simulink model "SMO_conventional"  (R2019b)
settings: Solver=VariableStepAuto  StartTime=0.0  StopTime=1  RelTol=1e-3
InitFcn:
  | run('MotorParamInit_1_5PMSM.m');
StopFcn:
  | %run('Calc_We_ThetaErr_Estimate_Harmonics.m');
values from neighbouring files (symbols this model uses):
  Ibase = 2*Pbase/Vbase/3    [MotorParamInit_1_5PMSM.m]
  J = 0.01    [MotorParamInit_1_5PMSM.m]
  KiPLL = 2*pi*fPIPLL*KpPLL    (= 209.439510239)    [MotorParamInit_1_5PMSM.m]
  KpCRd = 1.04    [MotorParamInit_1_5PMSM.m]
  KpCRq = 1.04    [MotorParamInit_1_5PMSM.m]
  KpPLL = 2*pi*fcutPLL/Webase    (= 1.66666666667)    [MotorParamInit_1_5PMSM.m]
  KpSR = 5.51    [MotorParamInit_1_5PMSM.m]
  Ld = 65.13e-3    (= 0.06513)    [MotorParamInit_1_5PMSM.m]
  LdPU = Ld/Lbase    [MotorParamInit_1_5PMSM.m]
  Lq = 120e-3    (= 0.12)    [MotorParamInit_1_5PMSM.m]
  LqPU = Lq/Lbase    [MotorParamInit_1_5PMSM.m]
  Np = 2    [MotorParamInit_1_5PMSM.m]
  PhifPU = Phif/Phibase    [MotorParamInit_1_5PMSM.m]
  Rs = 6.569    [MotorParamInit_1_5PMSM.m]
  RsPU = Rs/Zbase    [MotorParamInit_1_5PMSM.m]
  TaoiCRd = 4e-3    (= 0.004)    [MotorParamInit_1_5PMSM.m]
  TaoiCRq = 4e-3    (= 0.004)    [MotorParamInit_1_5PMSM.m]
  TaoiSR = 80e-3    (= 0.08)    [MotorParamInit_1_5PMSM.m]
  TaoLPF = 1/fLPF/2/pi    (= 0.00159154943092)    [MotorParamInit_1_5PMSM.m]
  Tctrl = 1/fctrl    (= 0.0001)    [MotorParamInit_1_5PMSM.m]
  TctrlPU = Tctrl/Tbase    (= 0.0376991118431)    [MotorParamInit_1_5PMSM.m]
  Tembase = Pbase/Wmbase    (= 7.95774715459)    [MotorParamInit_1_5PMSM.m]
  Ts = 1e-6    (= 1e-06)    [MotorParamInit_1_5PMSM.m]
  Vbase = VN*sqrt(2)/sqrt(3)    [MotorParamInit_1_5PMSM.m]
  Webase = 2*pi*fN    (= 376.991118431)    [MotorParamInit_1_5PMSM.m]
  Wmbase = Webase/Np    (= 188.495559215)    [MotorParamInit_1_5PMSM.m]
undefined symbols (not defined in the file or in its folder): DiscIntNeverNeededParam
libraries: simulink x6, powerlib x5, powerlib_extras x1
settings Model: Creator=W002220B  LastModifiedBy=W002220B

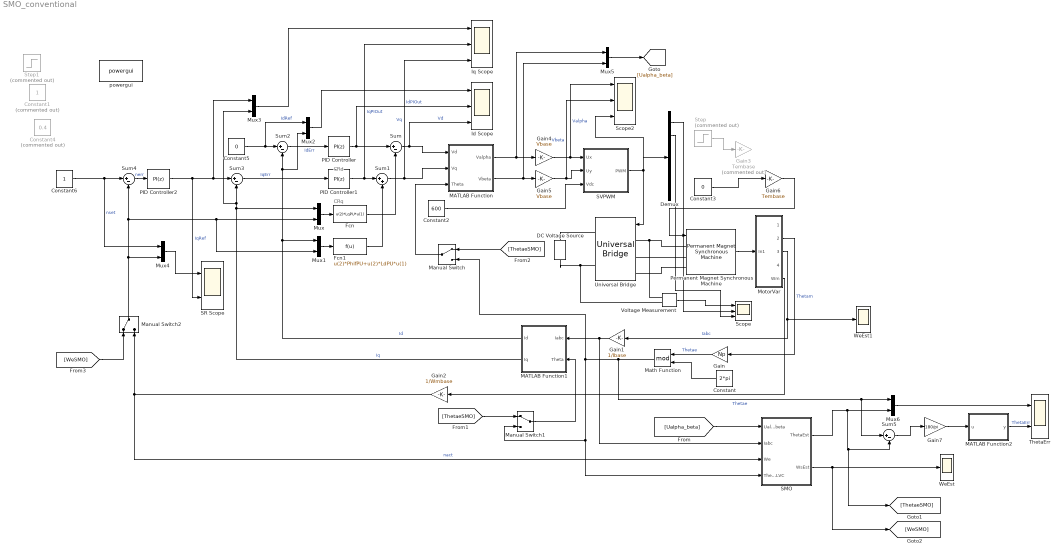
== system SMO_conventional ==
  note: CRd
  note: CRq
  Constant : Constant  Value=2*pi
  Constant1 : Constant  Commented=on
  Constant2 : Constant  Value=600
  Constant3 : Constant  Value=0
  Constant4 : Constant  Commented=on  Value=0.4
  Constant5 : Constant  Value=0
  Constant6 : Constant
  DC Voltage Source : powerlib/Electrical Sources/DC Voltage Source  Amplitude=600  Measurements=None
      settings: SourceProductName=Simscape Electrical
  Demux : Demux  Outputs=6
  Fcn : Fcn  Expr=u(2)*LqPU*u(1)
  Fcn1 : Fcn  Expr=u(2)*PhifPU+u(2)*LdPU*u(1)
  Gain : Gain  Gain=Np
  Gain1 : Gain  Gain=1/Ibase
  Gain2 : Gain  Gain=1/Wmbase
  Gain3 : Gain  Commented=on  Gain=Tembase
  Gain4 : Gain  Gain=Vbase
  Gain5 : Gain  Gain=Vbase
  Gain6 : Gain  Gain=Tembase
  Gain7 : Gain  Gain=180/pi
  Id Scope : Scope  NumInputPorts=3
  Iq Scope : Scope  NumInputPorts=3
  MATLAB Function : MATLAB Function  TreatAsAtomicUnit=on
  MATLAB Function1 : MATLAB Function  TreatAsAtomicUnit=on
  MATLAB Function2 : MATLAB Function  TreatAsAtomicUnit=on
  Manual Switch : ManualSwitch
  Manual Switch1 : ManualSwitch
  Manual Switch2 : ManualSwitch
  Math Function : Math  Operator=mod  SignedPower=off  SaturateOnIntegerOverflow=on
  MotorVar : Subsystem
  Mux{,1..6} (7 alike) : Mux  Inputs=2
  PID Controller : simulink/Continuous/PID Controller  Controller=PI  Form=Parallel  TimeDomain=Discrete-time  SampleTime=Tctrl  IntegratorMethod=Forward Euler  FilterMethod=Forward Euler  ControllerParametersSource=internal  P=KpCRd  I=KpCRd/TaoiCRd  D=0  UseFilter=on  N=100  TunerSelectOption=Transfer Function Based (PID Tuner App)  InitialConditionSource=internal  InitialConditionForIntegrator=0  InitialConditionForFilter=0  DifferentiatorICPrevScaledInput=0  ExternalReset=none  TrackingMode=off  Kt=1  LimitOutput=on  UpperSaturationLimit=0.5  LowerSaturationLimit=-0.5  LinearizeAsGain=on  AntiWindupMode=clamping  Kb=1  POutMin=[]  POutMax=[]  IOutMin=[]  IOutMax=[]  DOutMin=[]  DOutMax=[]  NOutMin=[]  NOutMax=[]  SumOutMin=[]  SumOutMax=[]  SaturationOutMin=[]  SaturationOutMax=[]  PParamMin=[]  PParamMax=[]  IParamMin=[]  IParamMax=[]  DParamMin=[]  DParamMax=[]  NParamMin=[]  NParamMax=[]  KbParamMin=[]  KbParamMax=[]  KtParamMin=[]  KtParamMax=[]  KbOutMin=[]  KbOutMax=[]  KtOutMin=[]  KtOutMax=[]  IntegratorOutMin=[]  IntegratorOutMax=[]  FilterOutMin=[]  FilterOutMax=[]  SumI1OutMin=[]  SumI1OutMax=[]  SumI2OutMin=[]  SumI2OutMax=[]  SumI3OutMin=[]  SumI3OutMax=[]  SumI4OutMin=[]  SumI4OutMax=[]  SumDOutMin=[]  SumDOutMax=[]  DifferentiatorOutMin=[]  DifferentiatorOutMax=[]  FilterDiffOutCoefMin=[]  FilterDiffOutCoefMax=[]  ReciprocalOutMin=[]  ReciprocalOutMax=[]  SumDenOutMin=[]  SumDenOutMax=[]  SumNumOutMin=[]  SumNumOutMax=[]  DivideOutMin=[]  DivideOutMax=[]  IntegratorContinuousStateAttributes=''  IntegratorStateMustResolveToSignalObject=off  IntegratorRTWStateStorageClass=Auto  FilterContinuousStateAttributes=''  FilterStateMustResolveToSignalObject=off  FilterRTWStateStorageClass=Auto  ParallelPVariant=InternalParameters  IdealPVariant=Disabled  IVariant=InternalParameters  DVariant=Disabled  IntegratorVariant=Discrete  SatVariant=Enabled  AWVariant=DiscClampingParallel  PCopyVariant=Disabled  TRVariant=Disabled  FdbkBlocksVariant=Forward  IdealPFdbkVariant=Disabled  SatFdbkVariant=Disabled  DerivativeFilterVariant=Disabled  NVariant=Disabled  NCopyVariant=Disabled_SignalSpec  FilterICVariant=Disabled  IntegratorICVariant=InternalICs  ExternalResetVariant=Disabled  TRSumVariant=Passthrough  SumFdbkVariant=Disabled  SumVariant=Sum_PI
  PID Controller1 : simulink/Continuous/PID Controller  Controller=PI  Form=Parallel  TimeDomain=Discrete-time  SampleTime=Tctrl  IntegratorMethod=Forward Euler  FilterMethod=Forward Euler  ControllerParametersSource=internal  P=KpCRq  I=KpCRq/TaoiCRq  D=0  UseFilter=on  N=100  TunerSelectOption=Transfer Function Based (PID Tuner App)  InitialConditionSource=internal  InitialConditionForIntegrator=0  InitialConditionForFilter=0  DifferentiatorICPrevScaledInput=0  ExternalReset=none  TrackingMode=off  Kt=1  LimitOutput=on  UpperSaturationLimit=0.5  LowerSaturationLimit=-0.5  LinearizeAsGain=on  AntiWindupMode=clamping  Kb=1  POutMin=[]  POutMax=[]  IOutMin=[]  IOutMax=[]  DOutMin=[]  DOutMax=[]  NOutMin=[]  NOutMax=[]  SumOutMin=[]  SumOutMax=[]  SaturationOutMin=[]  SaturationOutMax=[]  PParamMin=[]  PParamMax=[]  IParamMin=[]  IParamMax=[]  DParamMin=[]  DParamMax=[]  NParamMin=[]  NParamMax=[]  KbParamMin=[]  KbParamMax=[]  KtParamMin=[]  KtParamMax=[]  KbOutMin=[]  KbOutMax=[]  KtOutMin=[]  KtOutMax=[]  IntegratorOutMin=[]  IntegratorOutMax=[]  FilterOutMin=[]  FilterOutMax=[]  SumI1OutMin=[]  SumI1OutMax=[]  SumI2OutMin=[]  SumI2OutMax=[]  SumI3OutMin=[]  SumI3OutMax=[]  SumI4OutMin=[]  SumI4OutMax=[]  SumDOutMin=[]  SumDOutMax=[]  DifferentiatorOutMin=[]  DifferentiatorOutMax=[]  FilterDiffOutCoefMin=[]  FilterDiffOutCoefMax=[]  ReciprocalOutMin=[]  ReciprocalOutMax=[]  SumDenOutMin=[]  SumDenOutMax=[]  SumNumOutMin=[]  SumNumOutMax=[]  DivideOutMin=[]  DivideOutMax=[]  IntegratorContinuousStateAttributes=''  IntegratorStateMustResolveToSignalObject=off  IntegratorRTWStateStorageClass=Auto  FilterContinuousStateAttributes=''  FilterStateMustResolveToSignalObject=off  FilterRTWStateStorageClass=Auto  ParallelPVariant=InternalParameters  IdealPVariant=Disabled  IVariant=InternalParameters  DVariant=Disabled  IntegratorVariant=Discrete  SatVariant=Enabled  AWVariant=DiscClampingParallel  PCopyVariant=Disabled  TRVariant=Disabled  FdbkBlocksVariant=Forward  IdealPFdbkVariant=Disabled  SatFdbkVariant=Disabled  DerivativeFilterVariant=Disabled  NVariant=Disabled  NCopyVariant=Disabled_SignalSpec  FilterICVariant=Disabled  IntegratorICVariant=InternalICs  ExternalResetVariant=Disabled  TRSumVariant=Passthrough  SumFdbkVariant=Disabled  SumVariant=Sum_PI
  PID Controller2 : simulink/Continuous/PID Controller  Controller=PI  Form=Parallel  TimeDomain=Discrete-time  SampleTime=Tctrl  IntegratorMethod=Forward Euler  FilterMethod=Forward Euler  ControllerParametersSource=internal  P=KpSR  I=KpSR/TaoiSR  D=0  UseFilter=on  N=100  TunerSelectOption=Transfer Function Based (PID Tuner App)  InitialConditionSource=internal  InitialConditionForIntegrator=0  InitialConditionForFilter=0  DifferentiatorICPrevScaledInput=0  ExternalReset=none  TrackingMode=off  Kt=1  LimitOutput=on  UpperSaturationLimit=2  LowerSaturationLimit=-2  LinearizeAsGain=on  AntiWindupMode=clamping  Kb=1  POutMin=[]  POutMax=[]  IOutMin=[]  IOutMax=[]  DOutMin=[]  DOutMax=[]  NOutMin=[]  NOutMax=[]  SumOutMin=[]  SumOutMax=[]  SaturationOutMin=[]  SaturationOutMax=[]  PParamMin=[]  PParamMax=[]  IParamMin=[]  IParamMax=[]  DParamMin=[]  DParamMax=[]  NParamMin=[]  NParamMax=[]  KbParamMin=[]  KbParamMax=[]  KtParamMin=[]  KtParamMax=[]  KbOutMin=[]  KbOutMax=[]  KtOutMin=[]  KtOutMax=[]  IntegratorOutMin=[]  IntegratorOutMax=[]  FilterOutMin=[]  FilterOutMax=[]  SumI1OutMin=[]  SumI1OutMax=[]  SumI2OutMin=[]  SumI2OutMax=[]  SumI3OutMin=[]  SumI3OutMax=[]  SumI4OutMin=[]  SumI4OutMax=[]  SumDOutMin=[]  SumDOutMax=[]  DifferentiatorOutMin=[]  DifferentiatorOutMax=[]  FilterDiffOutCoefMin=[]  FilterDiffOutCoefMax=[]  ReciprocalOutMin=[]  ReciprocalOutMax=[]  SumDenOutMin=[]  SumDenOutMax=[]  SumNumOutMin=[]  SumNumOutMax=[]  DivideOutMin=[]  DivideOutMax=[]  IntegratorContinuousStateAttributes=''  IntegratorStateMustResolveToSignalObject=off  IntegratorRTWStateStorageClass=Auto  FilterContinuousStateAttributes=''  FilterStateMustResolveToSignalObject=off  FilterRTWStateStorageClass=Auto  ParallelPVariant=InternalParameters  IdealPVariant=Disabled  IVariant=InternalParameters  DVariant=Disabled  IntegratorVariant=Discrete  SatVariant=Enabled  AWVariant=DiscClampingParallel  PCopyVariant=Disabled  TRVariant=Disabled  FdbkBlocksVariant=Forward  IdealPFdbkVariant=Disabled  SatFdbkVariant=Disabled  DerivativeFilterVariant=Disabled  NVariant=Disabled  NCopyVariant=Disabled_SignalSpec  FilterICVariant=Disabled  IntegratorICVariant=InternalICs  ExternalResetVariant=Disabled  TRSumVariant=Passthrough  SumFdbkVariant=Disabled  SumVariant=Sum_PI
      settings: AttributesFormatString=SR
  Permanent Magnet Synchronous Machine : powerlib/Machines/Permanent Magnet Synchronous Machine  NbPhases=3  FluxDistribution=Sinusoidal  RotorType=Salient-pole  MechanicalLoad=Torque Tm  PresetModel=No  ShowDetailedParameters=on  MeasurementBus=off  Resistance=Rs  Inductance=8.5e-3  dqInductances=[Ld,Lq]  La=0.000395  MachineConstant=Flux linkage established by magnets (V.s)  Flux=Phif  VoltageCst=241.202  TorqueCst=1.9947  Flat=120  Mechanical=[J 0.0004924 Np 0]  PolePairs=4  InitialConditions=[0,0, 0,0]  InitialConditions5ph=[0 0 0 0 0 0]  RefAngle=Aligned with phase A axis (original Park)  IterativeDiscreteModel=Trapezoidal non iterative  TsBlock=-1  TsPowergui=0
  SMO : Subsystem
  SR Scope : Scope  NumInputPorts=2
  SVPWM : Subsystem  mask{DT=0e-6}
      mask prompts: DT "Dead Time (s)"
  Scope : Scope  NumInputPorts=3
  Scope2 : Scope  NumInputPorts=3
  Step : Step  Commented=on  SampleTime=0
  Step1 : Step  Commented=on  Before=0.2  After=0.3  SampleTime=0
  Sum{,2..5} (5 alike) : Sum  Inputs=|+-
  Sum1 : Sum  Inputs=|++
  ThetaErr : Scope  NumInputPorts=2
  Universal Bridge : powerlib/Power Electronics/Universal Bridge  Arms=3  SnubberResistance=1e5  SnubberCapacitance=inf  Device=MOSFET / Diodes  Ron=1e-3  Lon=0  ForwardVoltages="[  0  0  ]"  ForwardVoltage=0  GTOparameters=[ 10e-6 , 20e-6 ]  IGBTparameters=[ 1e-6 , 2e-6 ]  Measurements=None  Measurements_2=None  converterType=Rectifier
      settings: SourceProductName=Simscape Electrical
  Voltage Measurement : powerlib/Measurements/Voltage Measurement  PhasorSimulation=off  OutputType=Complex  PSBequivalent=0
      settings: SourceProductName=Simscape Electrical
  WeEst : Scope
  WeEst1 : Scope
  powergui : powerlib/powergui  Priority=1  SimulationMode=Discrete  SampleTime=Ts  frequency=60  Iterations=50  frequencyindice=0  Pbase=100e6  ErrMax=1e-4  UnitsV=kV  UnitsW=MW  buscounter=0  FunctionMessages=off  echomessages=off  EnableUseOfTLC=off  CurrentSourceSwitches=off  DisableSnubberDevices=off  DisableRonSwitches=off  DisableVfSwitches=off  DisplayEquations=off  AutomaticDiscreteSolvers=off  SolverType=Tustin/Backward Euler (TBE)  Interpol=off  ExternalGateDelay=off  methode=off  Ts=100  x0status=blocks  SPID=on  SwTol=0  HookPort=off  NonlinearTolerance=1e-4  nMaxIteration=100  ContinueOnMaxIteration=off  RestoreLinks=warning  ResistiveCurrentMeasurement=off  Frange=[0:2:500]  Ylog=off  Xlog=on  ShowGrid=off  save=off  variable=ZData  structure=0  ZoomFFT=off  StartTime=0.0  cycles=1  DisplayStyle=1  fundamental=60  FreqAxis=off  MaxFrequency=1000  frequencyindicesteady=1  RmsSteady=1  display=off
      settings: SourceProductName=Simscape Electrical
  wires:
  SVPWM/1(PWM) -> Universal Bridge/1, Demux/1, Scope2/3
  MATLAB Function/1(Valpha) -> Mux5/1, Gain4/1
  Sum/1 -> Id Scope/3, MATLAB Function/1(Vd)  "Vd"
  Sum1/1 -> Iq Scope/3, MATLAB Function/2(Vq)  "Vq"
  PID Controller/1 -> Id Scope/2, Sum/1  "IdPIOut"
  PID Controller1/1 -> Iq Scope/2, Sum1/1  "IqPIOut"
  Sum2/1 -> PID Controller/1  "IdErr"
  Constant5/1 -> Mux2/1, Sum2/1  "IdRef"
  Sum3/1 -> PID Controller1/1  "IqErr"
  Permanent Magnet Synchronous Machine/1 -> MotorVar/1(In1)
  Math Function/1 -> Sum5/1, Mux6/1, Manual Switch/2, Manual Switch1/2, SMO/4(ThetaCLVC)  "Thetae"
  MotorVar/2(Thetam) -> Gain/1  "Thetam"
  MATLAB Function1/1(Id) -> Mux1/1, Mux2/2, Sum2/2  "Id"
  MATLAB Function1/2(Iq) -> Mux/1, Mux3/2, Sum3/2  "Iq"
  Gain1/1 -> SMO/2(Iabc), MATLAB Function1/1(Iabc)
  MotorVar/3(Iabc) -> WeEst1/1, Gain1/1  "Iabc"
  Sum4/1 -> PID Controller2/1  "nerr"
  MotorVar/5(Wm) -> Gain2/1
  Constant2/1 -> SVPWM/3(Vdc)
  Mux/1 -> Fcn/1
  Fcn/1 -> Sum/2
  Fcn1/1 -> Sum1/2
  Mux1/1 -> Fcn1/1
  MATLAB Function/2(Vbeta) -> Mux5/2, Gain5/1
  Gain4/1 -> Scope2/1, SVPWM/1(Ux)  "Valpha"
  Gain5/1 -> Scope2/2, SVPWM/2(Uy)  "Vbeta"
  Mux2/1 -> Id Scope/1
  Mux3/1 -> Iq Scope/1
  Mux4/1 -> SR Scope/1
  Gain2/1 -> Manual Switch2/2, SMO/3(We)  "nact"
  Step/1 -> Gain3/1
  Voltage Measurement/1 -> Scope/1
  Demux/1 -> Scope/2
  Demux/2 -> Scope/3
  PID Controller2/1 -> SR Scope/2, Mux3/1, Sum3/1  "IqRef"
  Constant6/1 -> Sum4/1, Mux4/1  "nset"
  Mux5/1 -> [Ualpha_beta]
  [Ualpha_beta] -> SMO/1(Ualpha_beta)
  SMO/1(ThetaEst) -> Mux6/2, [ThetaeSMO], Sum5/2
  Mux6/1 -> ThetaErr/1
  SMO/2(WsEst) -> [WeSMO], WeEst/1
  Gain/1 -> Math Function/1  "Thetae"
  Constant/1 -> Math Function/2
  Constant3/1 -> Gain6/1
  Gain6/1 -> Permanent Magnet Synchronous Machine/1
  Sum5/1 -> Gain7/1
  MATLAB Function2/1(y) -> ThetaErr/2  "ThetaErr"
  Gain7/1 -> MATLAB Function2/1(u)
  Manual Switch1/1 -> MATLAB Function1/2(Theta)
  [ThetaeSMO] -> Manual Switch/1
  Manual Switch/1 -> MATLAB Function/3(Theta)
  [ThetaeSMO] -> Manual Switch1/1
  Manual Switch2/1 -> Mux4/2, Mux1/2, Mux/2, Sum4/2
  [WeSMO] -> Manual Switch2/1
  connections:
  Permanent Magnet Synchronous Machine/LConn2 -- Universal Bridge/LConn2
  Permanent Magnet Synchronous Machine/LConn3 -- Universal Bridge/LConn3
  Permanent Magnet Synchronous Machine/LConn1 -- Voltage Measurement/LConn1 -- Universal Bridge/LConn1
  DC Voltage Source/LConn1 -- Voltage Measurement/LConn2 -- Universal Bridge/RConn2
  DC Voltage Source/RConn1 -- Universal Bridge/RConn1

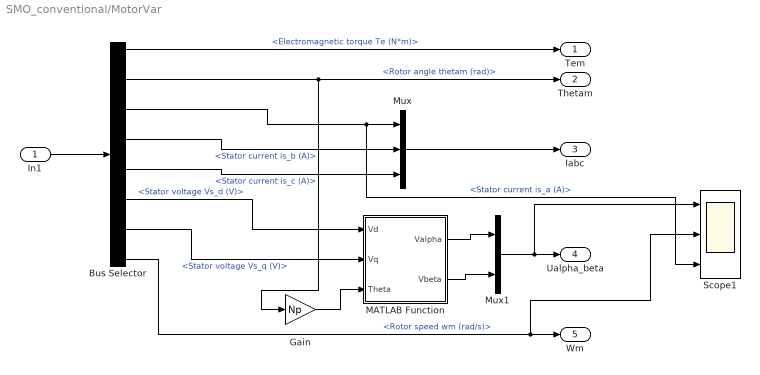
== system SMO_conventional/MotorVar ==
  In1 : Inport
  Bus Selector : BusSelector  OutputSignals=Electromagnetic torque Te (N*m),Rotor angle thetam (rad),Stator current is_a (A),Stator current is_b (A),Stator current is_c (A),Stator voltage Vs_d (V),Stator voltage Vs_q (V),Rotor speed wm (rad/s)
  Gain : Gain  Gain=Np
  MATLAB Function : MATLAB Function  TreatAsAtomicUnit=on
  Mux : Mux  Inputs=3
  Mux1 : Mux  Inputs=2
  Scope1 : Scope  NumInputPorts=3
  Tem : Outport
  Thetam : Outport  Port=2
  Iabc : Outport  Port=3
  Ualpha_beta : Outport  Port=4
  Wm : Outport  Port=5
  wires:
  In1/1 -> Bus Selector/1
  Bus Selector/1 -> Tem/1  "<Electromagnetic torque Te (N*m)>"
  Bus Selector/2 -> Gain/1, Thetam/1  "<Rotor angle thetam (rad)>"
  Bus Selector/3 -> Scope1/3, Mux/1  "<Stator current is_a (A)>"
  Mux/1 -> Iabc/1
  Bus Selector/6 -> MATLAB Function/1(Vd)  "<Stator voltage Vs_d (V)>"
  Bus Selector/7 -> MATLAB Function/2(Vq)  "<Stator voltage Vs_q (V)>"
  Gain/1 -> MATLAB Function/3(Theta)
  MATLAB Function/1(Valpha) -> Mux1/1
  MATLAB Function/2(Vbeta) -> Mux1/2
  Mux1/1 -> Scope1/1, Ualpha_beta/1
  Bus Selector/8 -> Scope1/2, Wm/1  "<Rotor speed wm (rad/s)>"
  Bus Selector/4 -> Mux/2  "<Stator current is_b (A)>"
  Bus Selector/5 -> Mux/3  "<Stator current is_c (A)>"

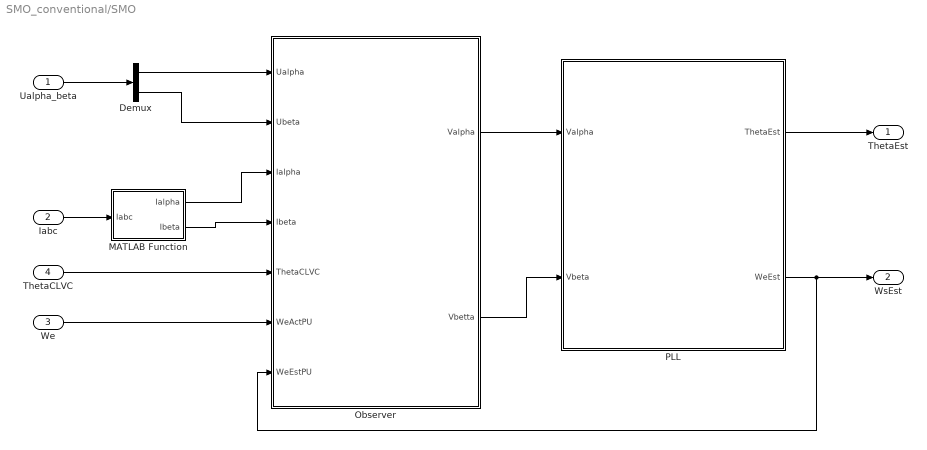
== system SMO_conventional/SMO ==
  Ualpha_beta : Inport
  Iabc : Inport  Port=2
  We : Inport  Port=3
  ThetaCLVC : Inport  Port=4
  Demux : Demux  Outputs=2
  MATLAB Function : MATLAB Function  TreatAsAtomicUnit=on
  Observer : Subsystem
  PLL : Subsystem
  ThetaEst : Outport
  WsEst : Outport  Port=2
  wires:
  Observer/1(Valpha) -> PLL/1(Valpha)
  Observer/2(Vbetta) -> PLL/2(Vbeta)
  PLL/1(ThetaEst) -> ThetaEst/1
  PLL/2(WeEst) -> Observer/7(WeEstPU), WsEst/1
  Iabc/1 -> MATLAB Function/1(Iabc)
  MATLAB Function/1(Ialpha) -> Observer/3(Ialpha)
  MATLAB Function/2(Ibeta) -> Observer/4(Ibeta)
  Ualpha_beta/1 -> Demux/1
  Demux/1 -> Observer/1(Ualpha)
  Demux/2 -> Observer/2(Ubeta)
  ThetaCLVC/1 -> Observer/5(ThetaCLVC)
  We/1 -> Observer/6(WeActPU)

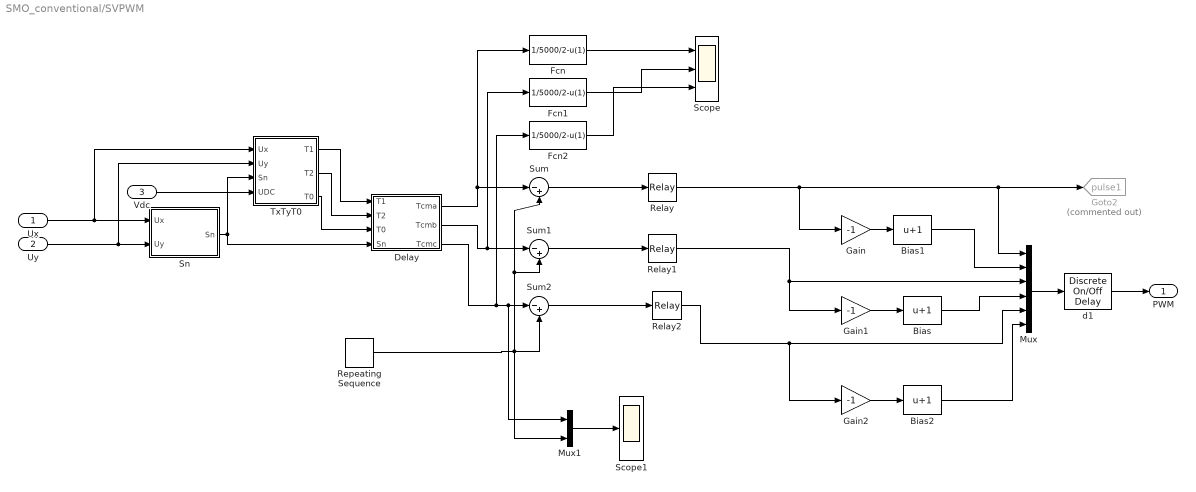
== system SMO_conventional/SVPWM ==
  Ux : Inport
  Uy : Inport  Port=2
  Vdc : Inport  Port=3
  Bias : Bias  Bias=1
  Bias1 : Bias  Bias=1
  Bias2 : Bias  Bias=1
  Delay : MATLAB Function  TreatAsAtomicUnit=on
  Fcn : Fcn  Expr=1/5000/2-u(1)
  Fcn1 : Fcn  Expr=1/5000/2-u(1)
  Fcn2 : Fcn  Expr=1/5000/2-u(1)
  Gain : Gain  Gain=-1
  Gain1 : Gain  Gain=-1
  Gain2 : Gain  Gain=-1
  Goto2 : Goto  Commented=on  GotoTag=pulse1  TagVisibility=global
  Mux : Mux  Inputs=6
  Mux1 : Mux  Inputs=2
  Relay : Relay  OnSwitchValue=0  OffSwitchValue=0
  Relay1 : Relay  OnSwitchValue=0  OffSwitchValue=0
  Relay2 : Relay  OnSwitchValue=0  OffSwitchValue=0
  Repeating Sequence : simulink/Sources/Repeating Sequence  rep_seq_t=[0 1/5000/2 1/5000]  rep_seq_y=[0 1/5000/2 0]
  Scope : Scope  NumInputPorts=3
  Scope1 : Scope
  Sn : MATLAB Function  TreatAsAtomicUnit=on
  Sum : Sum  Inputs=|-+
  Sum1 : Sum  Inputs=|-+
  Sum2 : Sum  Inputs=|-+
  TxTyT0 : MATLAB Function  TreatAsAtomicUnit=on
  d1 : powerlib_extras/Discrete  Control Blocks/Discrete On//Off Delay  type_delay=On delay  delay=DT  ic=0  Ts=Ts
      settings: SourceProductName=Simscape Electrical  SourceProductBaseCode=PS
  PWM : Outport
  wires:
  Delay/1(Tcma) -> Fcn/1, Sum/1
  Delay/2(Tcmb) -> Fcn1/1, Sum1/1
  Delay/3(Tcmc) -> Fcn2/1, Mux1/1, Sum2/1
  Repeating Sequence/1 -> Mux1/2, Sum2/2, Sum/2, Sum1/2
  Sum/1 -> Relay/1
  Sum2/1 -> Relay2/1
  Sum1/1 -> Relay1/1
  Relay1/1 -> Gain1/1, Mux/3
  Relay2/1 -> Gain2/1, Mux/5
  Sn/1(Sn) -> TxTyT0/3(Sn), Delay/4(Sn)
  TxTyT0/1(T1) -> Delay/1(T1)
  TxTyT0/2(T2) -> Delay/2(T2)
  TxTyT0/3(T0) -> Delay/3(T0)
  Gain1/1 -> Bias/1
  Gain/1 -> Bias1/1
  Gain2/1 -> Bias2/1
  Relay/1 -> Gain/1, Mux/1, Goto2/1
  Ux/1 -> Sn/1(Ux), TxTyT0/1(Ux)
  Uy/1 -> Sn/2(Uy), TxTyT0/2(Uy)
  Vdc/1 -> TxTyT0/4(UDC)
  Bias1/1 -> Mux/2
  Bias/1 -> Mux/4
  Bias2/1 -> Mux/6
  d1/1 -> PWM/1
  Mux/1 -> d1/1
  Fcn/1 -> Scope/1
  Fcn1/1 -> Scope/2
  Fcn2/1 -> Scope/3
  Mux1/1 -> Scope1/1

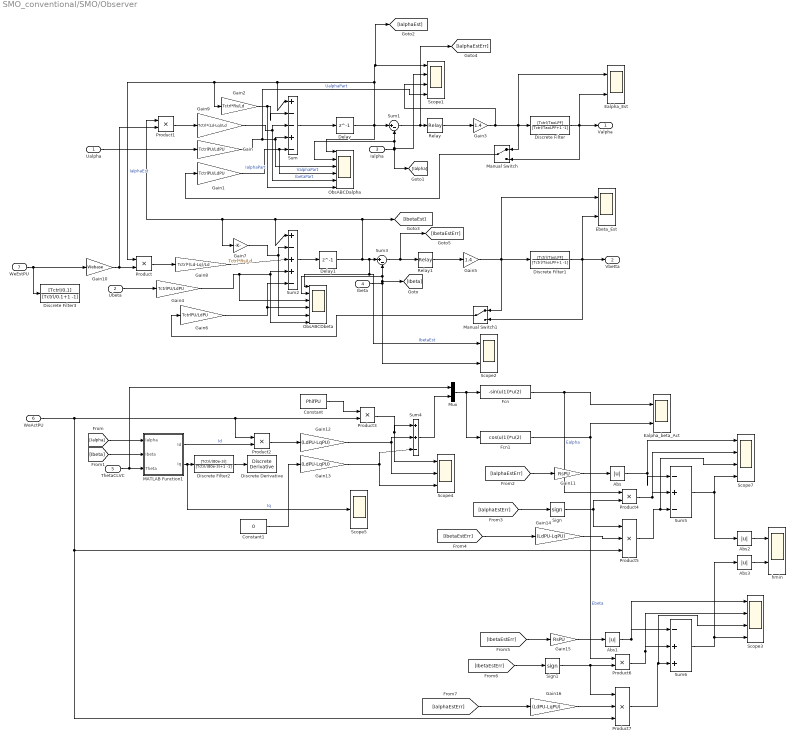
== system SMO_conventional/SMO/Observer ==
  Ualpha : Inport
  Ubeta : Inport  Port=2
  Ialpha : Inport  Port=3
  Ibeta : Inport  Port=4
  ThetaCLVC : Inport  Port=5
  WeActPU : Inport  Port=6
  WeEstPU : Inport  Port=7
  Abs{,1..3} (4 alike) : Abs
  Constant : Constant  Value=PhifPU
  Constant1 : Constant  Value=0
  Delay : Delay  DelayLength=1  InitialCondition=0  SampleTime=Tctrl
  Delay1 : Delay  DelayLength=1  InitialCondition=0  SampleTime=Tctrl
  Discrete Derivative : simulink/Discrete/Discrete Derivative  gainval=5  ICPrevScaledInput=0.0  OutMin=[]  OutMax=[]  OutDataType=fixdt(1, 16)  OutScaling=2^-10  DoSatur=off
  Discrete Filter : DiscreteFilter  Numerator=[Tctrl/TaoLPF]  Denominator=[Tctrl/TaoLPF+1 -1]  SampleTime=Tctrl
  Discrete Filter1 : DiscreteFilter  Numerator=[Tctrl/TaoLPF]  Denominator=[Tctrl/TaoLPF+1 -1]  SampleTime=Tctrl
  Discrete Filter2 : DiscreteFilter  Numerator=[Tctrl/(80e-3)]  Denominator=[Tctrl/(80e-3)+1 -1]
  Discrete Filter3 : DiscreteFilter  Numerator=[Tctrl/0.1]  Denominator=[Tctrl/0.1+1 -1]  SampleTime=Tctrl
  Ealpha_Est : Scope  NumInputPorts=2
  Ealpha_beta_Act : Scope  NumInputPorts=2
  Ebeta_Est : Scope  NumInputPorts=2
  Fcn : Fcn  Expr=-sin(u(1))*u(2)
  Fcn1 : Fcn  Expr=cos(u(1))*u(2)
  Gain{,1,4,6} (4 alike) : Gain  Gain=TctrlPU/LdPU
  Gain10 : Gain  Gain=Webase
  Gain11 : Gain  Gain=RsPU
  Gain{12..14,16} (4 alike) : Gain  Gain=(LdPU-LqPU)
  Gain15 : Gain  Gain=RsPU
  Gain2 : Gain  Gain=Tctrl*Rs/Ld
  Gain3 : Gain  Gain=1.4
  Gain5 : Gain  Gain=1.4
  Gain7 : Gain  Gain=Tctrl*Rs/Ld
  Gain8 : Gain  Gain=Tctrl*(Ld-Lq)/Ld
  Gain9 : Gain  Gain=Tctrl*(Ld-Lq)/Ld
  MATLAB Function1 : MATLAB Function  TreatAsAtomicUnit=on
  Manual Switch : ManualSwitch
  Manual Switch1 : ManualSwitch
  Mux : Mux  Inputs=2
  ObsABCDalpha : Scope  NumInputPorts=6
  ObsABCDbeta : Scope  NumInputPorts=6
  Product{,1..4,6} (6 alike) : Product
  Product5 : Product  Inputs=3
  Product7 : Product  Inputs=3
  Relay : Relay  OnSwitchValue=0  OffSwitchValue=0  OffOutputValue=-1
  Relay1 : Relay  OnSwitchValue=0  OffSwitchValue=0  OffOutputValue=-1
  Scope1 : Scope  NumInputPorts=4
  Scope2 : Scope  NumInputPorts=2
  Scope3 : Scope  NumInputPorts=4
  Scope4 : Scope  NumInputPorts=3
  Scope5 : Scope  NumInputPorts=3
  Scope7 : Scope  NumInputPorts=4
  Sign : Signum
  Sign1 : Signum
  Sum : Sum  Inputs=|+--+-
  Sum1 : Sum  Inputs=|+-
  Sum2 : Sum  Inputs=|+-++-
  Sum3 : Sum  Inputs=|+-
  Sum4 : Sum  Inputs=|++-
  Sum5 : Sum  Inputs=|-+-
  Sum6 : Sum  Inputs=|-++
  hmin : Scope  NumInputPorts=2
  Valpha : Outport
  Vbetta : Outport  Port=2
  wires:
  Ualpha/1 -> Gain/1
  Gain/1 -> Scope1/4, ObsABCDalpha/3, Sum/4  "UalphaPart"
  Gain1/1 -> ObsABCDalpha/4, Sum/5  "ValphaPart"
  Sum/1 -> Delay/1
  Delay/1 -> ObsABCDalpha/1, Sum1/1, [IalphaEst], Scope1/1, Sum/1, Product/1, Gain2/1  "IalphaEst"
  Relay/1 -> Gain3/1
  Gain3/1 -> Scope1/3, Ealpha_Est/1, Manual Switch/1, Discrete Filter/1
  Gain2/1 -> ObsABCDalpha/6, Sum/2  "IalphaPart"
  Sum1/1 -> [IalphaEstErr], Relay/1
  Ialpha/1 -> Scope1/2, ObsABCDalpha/2, Sum1/2, [Ialpha]
  Ubeta/1 -> Gain4/1
  Gain4/1 -> ObsABCDbeta/3, ObsABCDbeta/6, Sum2/4
  Sum2/1 -> Delay1/1
  Ibeta/1 -> [Ibeta], ObsABCDbeta/2, Sum3/2, Scope2/2
  Delay1/1 -> ObsABCDbeta/1, Scope2/1, Sum3/1, Sum2/1, Product1/1, Gain7/1, [IbetaEst]  "IbetaEst"
  Sum3/1 -> [IbetaEstErr], Relay1/1
  Relay1/1 -> Gain5/1
  Gain5/1 -> Ebeta_Est/1, Manual Switch1/1, Discrete Filter1/1
  Gain6/1 -> ObsABCDbeta/4, Sum2/5
  Gain7/1 -> ObsABCDbeta/5, Sum2/2
  Gain8/1 -> Sum2/3
  Product/1 -> Gain8/1
  Product1/1 -> Gain9/1
  Gain9/1 -> ObsABCDalpha/5, Sum/3  "IbetaPart"
  Discrete Filter/1 -> Valpha/1, Ealpha_Est/2, Manual Switch/2
  Discrete Filter1/1 -> Vbetta/1, Ebeta_Est/2, Manual Switch1/2
  Manual Switch/1 -> Gain1/1
  Manual Switch1/1 -> Gain6/1
  WeActPU/1 -> Product7/3, Product5/3, Product2/1, Product3/2
  Gain10/1 -> Product1/2, Product/2
  ThetaCLVC/1 -> Mux/1, MATLAB Function1/3(Theta)
  [Ibeta] -> MATLAB Function1/2(Ibeta)
  [Ialpha] -> MATLAB Function1/1(Ialpha)
  MATLAB Function1/1(Id) -> Product2/2  "Id"
  Product2/1 -> Gain12/1
  Constant/1 -> Product3/1
  Gain12/1 -> Scope4/2, Sum4/2
  Gain13/1 -> Scope4/3, Sum4/3
  Product3/1 -> Scope4/1, Sum4/1
  Sum4/1 -> Mux/2
  Mux/1 -> Fcn1/1, Fcn/1
  Fcn/1 -> Product4/1, Ealpha_beta_Act/1  "Ealpha"
  Fcn1/1 -> Ealpha_beta_Act/2, Product6/1  "Ebeta"
  MATLAB Function1/2(Iq) -> Scope5/2, Discrete Filter2/1  "Iq"
  Discrete Filter2/1 -> Discrete Derivative/1
  Constant1/1 -> Gain13/1
  [IalphaEstErr] -> Gain11/1
  Product4/1 -> Scope7/2, Sum5/2
  [IalphaEstErr] -> Sign/1
  Sign/1 -> Product5/1, Product4/2
  Product5/1 -> Scope7/3, Sum5/3
  [IbetaEstErr] -> Gain14/1
  Gain14/1 -> Product5/2
  Gain11/1 -> Abs/1
  Abs/1 -> Scope7/1, Sum5/1
  Gain15/1 -> Abs1/1
  [IbetaEstErr] -> Gain15/1
  Abs1/1 -> Scope3/1, Sum6/1
  Product6/1 -> Scope3/2, Sum6/2
  [IbetaEstErr] -> Sign1/1
  Sign1/1 -> Product7/1, Product6/2
  Product7/1 -> Scope3/3, Sum6/3
  [IalphaEstErr] -> Gain16/1
  Gain16/1 -> Product7/2
  Abs3/1 -> hmin/2
  Abs2/1 -> hmin/1
  Sum5/1 -> Scope7/4, Abs2/1
  Sum6/1 -> Scope3/4, Abs3/1
  WeEstPU/1 -> Discrete Filter3/1, Gain10/1

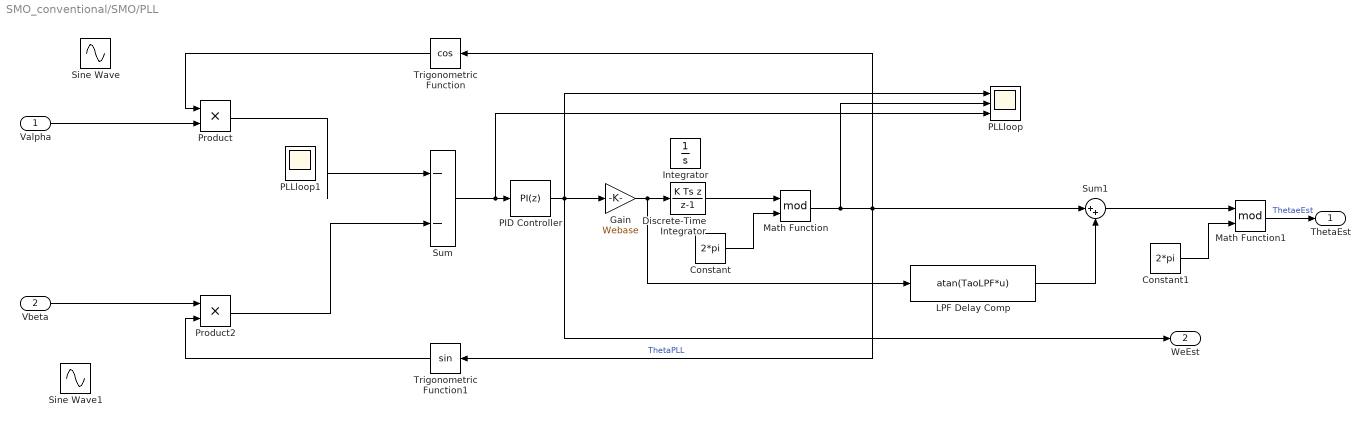
== system SMO_conventional/SMO/PLL ==
  Valpha : Inport
  Vbeta : Inport  Port=2
  Constant : Constant  Value=2*pi
  Constant1 : Constant  Value=2*pi
  Discrete-Time Integrator : DiscreteIntegrator  IntegratorMethod=Integration: Backward Euler  gainval=1  SampleTime=Tctrl  ICPrevOutput=DiscIntNeverNeededParam  ICPrevScaledInput=DiscIntNeverNeededParam
  Gain : Gain  Gain=Webase
  Integrator : Integrator
  LPF Delay Comp : Fcn  Expr=atan(TaoLPF*u)
  Math Function : Math  Operator=mod  SignedPower=off  SaturateOnIntegerOverflow=on
  Math Function1 : Math  Operator=mod  SignedPower=off  SaturateOnIntegerOverflow=on
  PID Controller : simulink/Continuous/PID Controller  Controller=PI  Form=Parallel  TimeDomain=Discrete-time  SampleTime=Tctrl  IntegratorMethod=Forward Euler  FilterMethod=Forward Euler  ControllerParametersSource=internal  P=KpPLL  I=KiPLL  D=0  UseFilter=on  N=100  TunerSelectOption=Transfer Function Based (PID Tuner App)  InitialConditionSource=internal  InitialConditionForIntegrator=0  InitialConditionForFilter=0  DifferentiatorICPrevScaledInput=0  ExternalReset=none  TrackingMode=off  Kt=1  LimitOutput=on  UpperSaturationLimit=4.4  LowerSaturationLimit=-4.4  LinearizeAsGain=on  AntiWindupMode=clamping  Kb=1  POutMin=[]  POutMax=[]  IOutMin=[]  IOutMax=[]  DOutMin=[]  DOutMax=[]  NOutMin=[]  NOutMax=[]  SumOutMin=[]  SumOutMax=[]  SaturationOutMin=[]  SaturationOutMax=[]  PParamMin=[]  PParamMax=[]  IParamMin=[]  IParamMax=[]  DParamMin=[]  DParamMax=[]  NParamMin=[]  NParamMax=[]  KbParamMin=[]  KbParamMax=[]  KtParamMin=[]  KtParamMax=[]  KbOutMin=[]  KbOutMax=[]  KtOutMin=[]  KtOutMax=[]  IntegratorOutMin=[]  IntegratorOutMax=[]  FilterOutMin=[]  FilterOutMax=[]  SumI1OutMin=[]  SumI1OutMax=[]  SumI2OutMin=[]  SumI2OutMax=[]  SumI3OutMin=[]  SumI3OutMax=[]  SumI4OutMin=[]  SumI4OutMax=[]  SumDOutMin=[]  SumDOutMax=[]  DifferentiatorOutMin=[]  DifferentiatorOutMax=[]  FilterDiffOutCoefMin=[]  FilterDiffOutCoefMax=[]  ReciprocalOutMin=[]  ReciprocalOutMax=[]  SumDenOutMin=[]  SumDenOutMax=[]  SumNumOutMin=[]  SumNumOutMax=[]  DivideOutMin=[]  DivideOutMax=[]  IntegratorContinuousStateAttributes=''  IntegratorStateMustResolveToSignalObject=off  IntegratorRTWStateStorageClass=Auto  FilterContinuousStateAttributes=''  FilterStateMustResolveToSignalObject=off  FilterRTWStateStorageClass=Auto  ParallelPVariant=InternalParameters  IdealPVariant=Disabled  IVariant=InternalParameters  DVariant=Disabled  IntegratorVariant=Discrete  SatVariant=Enabled  AWVariant=DiscClampingParallel  PCopyVariant=Disabled  TRVariant=Disabled  FdbkBlocksVariant=Forward  IdealPFdbkVariant=Disabled  SatFdbkVariant=Disabled  DerivativeFilterVariant=Disabled  NVariant=Disabled  NCopyVariant=Disabled_SignalSpec  FilterICVariant=Disabled  IntegratorICVariant=InternalICs  ExternalResetVariant=Disabled  TRSumVariant=Passthrough  SumFdbkVariant=Disabled  SumVariant=Sum_PI
  PLLloop : Scope  NumInputPorts=3
  PLLloop1 : Scope  NumInputPorts=3
  Product : Product
  Product2 : Product
  Sine Wave : Sin  Frequency=50*2*pi  Phase=pi/2  SampleTime=0
  Sine Wave1 : Sin  Frequency=50*2*pi  SampleTime=0
  Sum : Sum  Inputs=|--
  Sum1 : Sum  Inputs=|++
  Trigonometric Function : Trigonometry  Operator=cos
  Trigonometric Function1 : Trigonometry
  ThetaEst : Outport
  WeEst : Outport  Port=2
  wires:
  Product/1 -> Sum/1
  Sum/1 -> PID Controller/1, PLLloop/3
  Discrete-Time Integrator/1 -> Math Function/1
  Product2/1 -> Sum/2
  Trigonometric Function/1 -> Product/1
  Trigonometric Function1/1 -> Product2/2
  Constant/1 -> Math Function/2
  Math Function/1 -> PLLloop/2, Trigonometric Function1/1, Sum1/1, Trigonometric Function/1  "ThetaPLL"
  PID Controller/1 -> WeEst/1, PLLloop/1, Gain/1
  Gain/1 -> LPF Delay Comp/1, Discrete-Time Integrator/1
  Valpha/1 -> Product/2
  Vbeta/1 -> Product2/1
  LPF Delay Comp/1 -> Sum1/2
  Constant1/1 -> Math Function1/2
  Sum1/1 -> Math Function1/1
  Math Function1/1 -> ThetaEst/1  "ThetaeEst"

== matlab function SMO_conventional/SVPWM/Sn ==
  data: Sn output; Ux input; Uy input
function Sn = S(Ux,Uy)
theta=atan2(Uy,Ux)*180/pi;
if theta>=0&&theta<60
    Sn=1;
elseif theta>=60&&theta<120
    Sn=2;
elseif theta>=120&&theta<180
    Sn=3;
elseif theta>=-180&&theta<-120
    Sn=4;
elseif theta>=-120&&theta<-60
    Sn=5;
else Sn=6;
end

== matlab function SMO_conventional/MATLAB Function ==
  data: Valpha output; Vd input; Vbeta output; Vq input; Theta input
function [Valpha, Vbeta] = fcn(Vd, Vq, Theta)
%#codegen

Valpha = Vd*cos(Theta) - Vq*sin(Theta);
Vbeta  = Vd*sin(Theta) + Vq*cos(Theta);

== matlab function SMO_conventional/SVPWM/TxTyT0 ==
  data: Ux input; Uy input; Sn input; T1 output; T2 output; T0 output; UDC input
function [T1,T2,T0]=T(Ux,Uy,Sn,UDC)
Ts=1/5000;
Udc=UDC;

X=sqrt(3)*Ts/Udc*Uy;
Y=sqrt(3)*Ts/2/Udc*(sqrt(3)*Ux+Uy);
Z=sqrt(3)*Ts/2/Udc*(-sqrt(3)*Ux+Uy);

if Sn==1
    T1=-Z;T2=X;
elseif Sn==2;
    T1=Z;T2=Y;
elseif Sn==3;
    T1=X;T2=-Y;
elseif Sn==4;
    T1=-X;T2=Z;
elseif Sn==5;
    T1=-Y;T2=-Z;
else T1=Y;T2=-X;
end
    
if T1+T2>Ts
    a=T1;b=T2;
    T1=a*Ts/(a+b);
    T2=b*Ts/(a+b);
end

T0=Ts-T1-T2;

== matlab function SMO_conventional/SVPWM/Delay ==
  data: T1 input; T2 input; T0 input; Tcma output; Tcmb output; Tcmc output; Sn input
function [Tcma,Tcmb,Tcmc]=D(T1,T2,T0,Sn)
T=1/5000;
ton1=0.25*T0;
ton2=ton1+T1/2;
ton3=ton2+T2/2;
if Sn==1
    Tcma=ton1;Tcmb=ton2;Tcmc=ton3;
elseif Sn==2;
    Tcma=ton2;Tcmb=ton1;Tcmc=ton3;
elseif Sn==3;
    Tcma=ton3;Tcmb=ton1;Tcmc=ton2;
elseif Sn==4;
    Tcma=ton3;Tcmb=ton2;Tcmc=ton1;
elseif Sn==5;
    Tcma=ton2;Tcmb=ton3;Tcmc=ton1;
else Tcma=ton1;Tcmb=ton3;Tcmc=ton2;
end

== matlab function SMO_conventional/MotorVar/MATLAB Function ==
  data: Valpha output; Vd input; Vbeta output; Vq input; Theta input
function [Valpha, Vbeta] = fcn(Vd, Vq, Theta)
%#codegen

Valpha = Vd*cos(Theta) - Vq*sin(Theta);
Vbeta  = Vd*sin(Theta) + Vq*cos(Theta);

== matlab function SMO_conventional/MATLAB Function1 ==
  data: Id output; Iabc input; Iq output; Theta input
function [Id, Iq] = fcn(Iabc,Theta)
%#codegen

Id =  Iabc(1)*cos(Theta) + Iabc(2)*cos(Theta-2*pi/3) + Iabc(3)*cos(Theta+2*pi/3);
Iq  = -Iabc(1)*sin(Theta) - Iabc(2)*sin(Theta-2*pi/3) - Iabc(3)*sin(Theta+2*pi/3);
Id = Id*2/3;
Iq = Iq*2/3;

== matlab function SMO_conventional/SMO/MATLAB Function ==
  data: Iabc input; Ialpha output; Ibeta output
function [Ialpha,Ibeta] = fcn(Iabc)
Ialpha = Iabc(1) - Iabc(2)/2 - Iabc(3)/2;
Ibeta  = sqrt(3)/2*(Iabc(2) - Iabc(3));

Ialpha = Ialpha*2/3;
Ibeta  = Ibeta *2/3;

== matlab function SMO_conventional/SMO/Observer/MATLAB Function1 ==
  data: Id output; Ialpha input; Ibeta input; Iq output; Theta input
function [Id, Iq] = fcn(Ialpha, Ibeta,Theta)
%#codegen

Id  =  Ialpha*cos(Theta) + Ibeta*sin(Theta);
Iq  = -Ialpha*sin(Theta) + Ibeta*cos(Theta);

== matlab function SMO_conventional/MATLAB Function2 ==
  data: u input; y output
function y = fcn(u)
y=mod(u,360);
y=y-floor(y/180)*360;
